simulink model "cascade_pid_model"  (R2018b)
settings: Solver=ode1  StartTime=0.0  StopTime=10.0  FixedStep=0.002  RelTol=1e-3  EnableMultiTasking=on
settings Model: Creator=Robert  LastModifiedBy=Robert

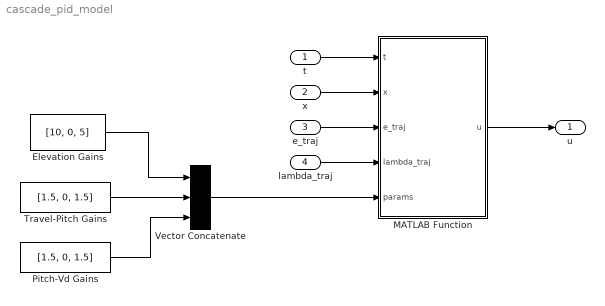
== system cascade_pid_model ==
  t : Inport  PortDimensions=1
  x : Inport  Port=2  PortDimensions=6
  e_traj : Inport  Port=3  PortDimensions=5
  lambda_traj : Inport  Port=4  PortDimensions=5
  Elevation Gains : Constant  Value=[10, 0, 5]
  MATLAB Function : MATLAB Function  TreatAsAtomicUnit=on
  Pitch-Vd Gains : Constant  Value=[1.5, 0, 1.5]
  Travel-Pitch Gains : Constant  Value=[1.5, 0, 1.5]
  Vector Concatenate : Concatenate  NumInputs=3
  u : Outport
  wires:
  Travel-Pitch Gains/1 -> Vector Concatenate/2
  Elevation Gains/1 -> Vector Concatenate/1
  Pitch-Vd Gains/1 -> Vector Concatenate/3
  Vector Concatenate/1 -> MATLAB Function/5(params)
  t/1 -> MATLAB Function/1(t)
  lambda_traj/1 -> MATLAB Function/4(lambda_traj)
  e_traj/1 -> MATLAB Function/3(e_traj)
  x/1 -> MATLAB Function/2(x)
  MATLAB Function/1(u) -> u/1

== matlab function cascade_pid_model/MATLAB Function ==
  data: t input; u output; x input; e_traj input; lambda_traj input; params input
function u = fcn(t, x, e_traj, lambda_traj, params)
    u = cascade_pid(t, x, e_traj, lambda_traj, params);
end
